simulink model "lidar_webcam_interpolation"  (Simulink 7.3)
settings: Solver=FixedStepDiscrete  StartTime=0.0  StopTime=inf  MaxStep=0.2  RelTol=1e-3
libraries: vipstatistics x1, simulink x1, dspstat3 x1, dspmtrx3 x1
settings Model: Creator=gclayton  LastModifiedBy=wildcat
settings DebuggingCC: InheritedTsInSrcMsg=none
settings RTWCC: SystemTargetFile=rlnx.tlc  GenCodeOnly=on  TemplateMakefile=rlnx_ubuntu.tmf  Description=Linux Real-Time Target  ProcessScript=rlnx_make_rtw_hook
settings RTWCC: CustomInclude=|
  | /usr/local/include/opencv/
  | /usr/local/include/
settings CodeAppCC: GenerateComments=off  SimulinkBlockComments=off
settings STFCustomTargetCC: ModelReferenceCompliant=off  MatFileLogging=on  SystemTargetFile=rlnx.tlc
settings GRTTargetCC: ModelReferenceCompliant=off  ParMdlRefBuildCompliant=off  CompOptLevelCompliant=off
settings CustomProperty: DataType=string  Value=-lm -ldl /usr/local/lib/libopencv_highgui.so.2.4 /usr/local/lib/libopencv_core.so.2.4 /usr/local/lib/libopencv_imgproc.so.2.4 -lc_urg -lc_urg_connection -lc_urg_system -lphidget21
settings EnumStrPairs: String=PC

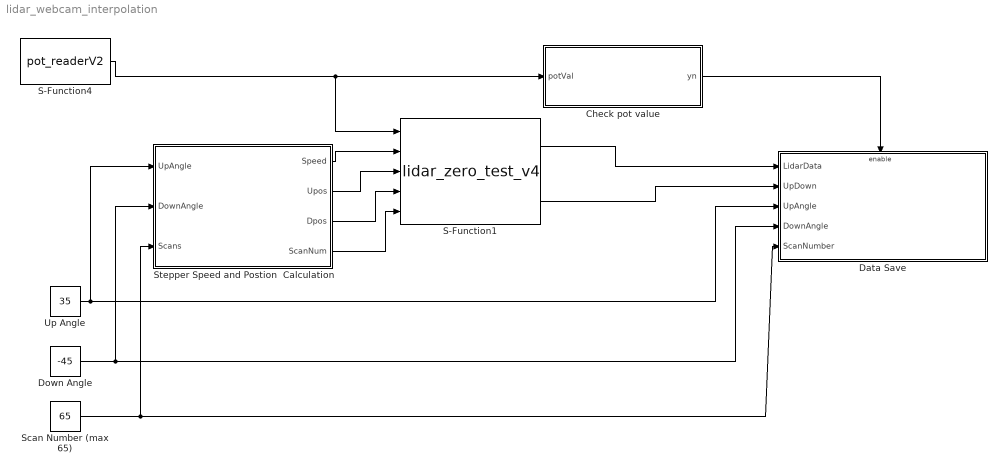
== system lidar_webcam_interpolation ==
  Check pot value : Stateflow chart  TreatAsAtomicUnit=on
  Data Save : Subsystem  TreatAsAtomicUnit=on
  Down Angle : Constant  Value=-45
  S-Function1 : S-Function  FunctionName=lidar_zero_test_v4  EnableBusSupport=off
  S-Function4 : S-Function  FunctionName=pot_readerV2  EnableBusSupport=off
  Scan Number (max 65) : Constant  Value=65
  Stepper Speed and Postion  Calculation : Stateflow chart  TreatAsAtomicUnit=on
  Up Angle : Constant  Value=35
  wires:
  S-Function4/1 -> S-Function1/1, Check pot value/1(potVal)
  Check pot value/1(yn) -> Data Save/Enable
  Scan Number (max 65)/1 -> Stepper Speed and Postion  Calculation/3(Scans), Data Save/5(ScanNumber)
  Down Angle/1 -> Stepper Speed and Postion  Calculation/2(DownAngle), Data Save/4(DownAngle)
  Up Angle/1 -> Stepper Speed and Postion  Calculation/1(UpAngle), Data Save/3(UpAngle)
  Stepper Speed and Postion  Calculation/1(Speed) -> S-Function1/2
  Stepper Speed and Postion  Calculation/2(Upos) -> S-Function1/3
  Stepper Speed and Postion  Calculation/3(Dpos) -> S-Function1/4
  Stepper Speed and Postion  Calculation/4(ScanNum) -> S-Function1/5
  S-Function1/1 -> Data Save/1(LidarData)
  S-Function1/2 -> Data Save/2(UpDown)

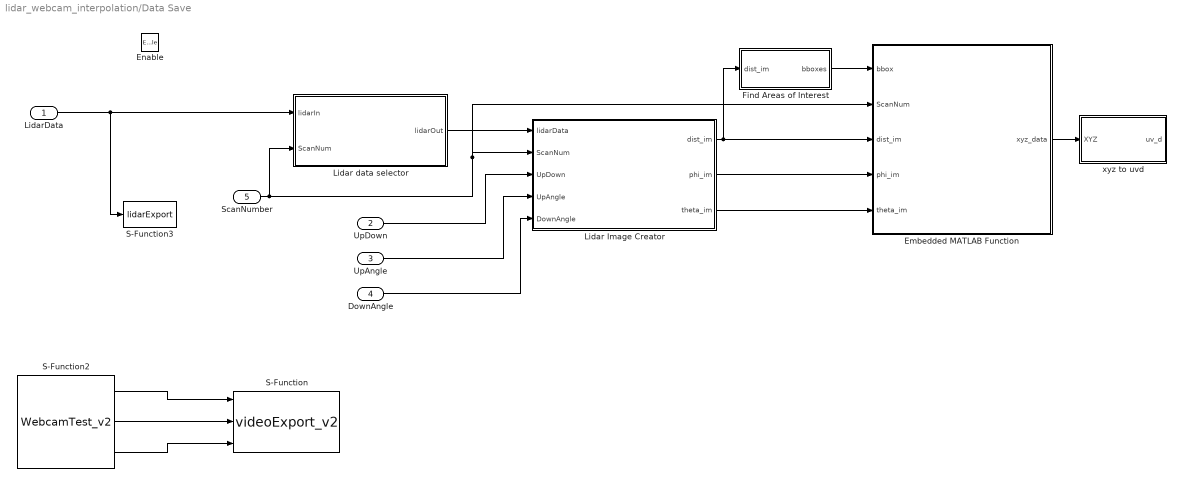
== system lidar_webcam_interpolation/Data Save ==
  LidarData : Inport
  UpDown : Inport  Port=2
  UpAngle : Inport  Port=3
  DownAngle : Inport  Port=4
  ScanNumber : Inport  Port=5
  Enable : EnablePort
  Embedded MATLAB Function : Stateflow chart  TreatAsAtomicUnit=on
  Find Areas of Interest : Subsystem
  Lidar Image Creator : Stateflow chart  TreatAsAtomicUnit=on
  Lidar data selector : Stateflow chart  TreatAsAtomicUnit=on
  S-Function : S-Function  FunctionName=videoExport_v2  EnableBusSupport=off
  S-Function2 : S-Function  FunctionName=WebcamTest_v2  EnableBusSupport=off
  S-Function3 : S-Function  FunctionName=lidarExport  EnableBusSupport=off
  xyz to uvd : Stateflow chart  TreatAsAtomicUnit=on
  wires:
  S-Function2/3 -> S-Function/3
  S-Function2/2 -> S-Function/2
  S-Function2/1 -> S-Function/1
  LidarData/1 -> S-Function3/1, Lidar data selector/1(lidarIn)
  ScanNumber/1 -> Lidar data selector/2(ScanNum), Lidar Image Creator/2(ScanNum), Embedded MATLAB Function/2(ScanNum)
  Lidar data selector/1(lidarOut) -> Lidar Image Creator/1(lidarData)
  UpDown/1 -> Lidar Image Creator/3(UpDown)
  UpAngle/1 -> Lidar Image Creator/4(UpAngle)
  DownAngle/1 -> Lidar Image Creator/5(DownAngle)
  Lidar Image Creator/1(dist_im) -> Embedded MATLAB Function/3(dist_im), Find Areas of Interest/1(dist_im)
  Lidar Image Creator/2(phi_im) -> Embedded MATLAB Function/4(phi_im)
  Lidar Image Creator/3(theta_im) -> Embedded MATLAB Function/5(theta_im)
  Find Areas of Interest/1(bboxes) -> Embedded MATLAB Function/1(bbox)
  Embedded MATLAB Function/1(xyz_data) -> xyz to uvd/1(XYZ)

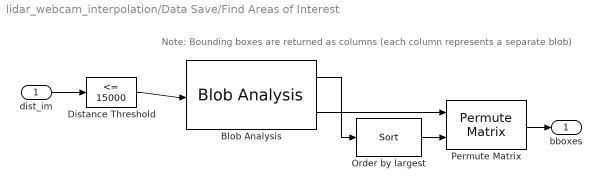
== system lidar_webcam_interpolation/Data Save/Find Areas of Interest ==
  note: Note: Bounding boxes are returned as columns (each column represents a separate blob)
  dist_im : Inport
  Blob Analysis : vipstatistics/Blob Analysis  Tag=vipblks_row_conv  area=on  centroid=off  bBox=on  majorAxis=off  minorAxis=off  angle=off  eccentricity=off  equivDiameterSq=off  extent=off  perimeter=off  maxBlobs=8  warnIfNumBlobsExceeded=on  isCount=off  useMinArea=off  minArea=0  useMaxArea=off  maxArea=intmax('uint32')  excludeBorderBlob=off  outDT=double  isOutVarDim=off  isFill=on  fillValues=-1  conn=8  isLabel=off  outputMode=Binary point scaling  outputWordLength=32  outputFracLength=16  firstCoeffMode=Binary point scaling  firstCoeffWordLength=16  firstCoeffFracLength=14  secondCoeffMode=Binary point scaling  secondCoeffWordLength=32  secondCoeffFracLength=16  accumMode=Binary point scaling  accumWordLength=32  accumFracLength=0  prodOutputMode=Binary point scaling  prodOutputWordLength=32  prodOutputFracLength=16  roundingMode=Floor  overflowMode=off
  Distance Threshold : simulink/Logic and Bit Operations/Compare To Constant  relop=<=  const=15000  OutDataTypeStr=boolean  ZeroCross=off
  Order by largest : dspstat3/Sort  otype=Index  dir=Descending  sortAlg=Quick sort  accumDataTypeStr=Inherit: Same as product output  accumLastDataTypeStr=Inherit: Same as product output  roundingMode=Floor  overflowMode=off
  Permute Matrix : dspmtrx3/Permute Matrix  mode=Columns  ZeroOneIdxMode=One-based  errmode=Clip index  checkDims=off
  bboxes : Outport
  wires:
  dist_im/1 -> Distance Threshold/1
  Distance Threshold/1 -> Blob Analysis/1
  Blob Analysis/2 -> Permute Matrix/1
  Order by largest/1 -> Permute Matrix/2
  Blob Analysis/1 -> Order by largest/1
  Permute Matrix/1 -> bboxes/1

== matlab function Stepper Speed and Postion Calculation ==
  data: UpAngle input double; Speed output double; DownAngle input double; Scans input double; Upos output double; Dpos output double; ScanNum output double
function [Speed,Upos,Dpos,ScanNum] = stepper_calc(UpAngle,DownAngle,Scans)

% This function inputs desired positive and negative scan angles
% and desired number of scans and outputs results positions for
% the stepper and the required speed of the stepper motor to properly
% move so the desired number of scans is obtained over the course of
% the motion of the stepper

% Scan Number requires no change
ScanNum = Scans;

% Transformation of angle to stepper position obtained from stepper calibration
% Output must be an integer
% 57 is added or subtracted due to wobble of gimbal system
Upos = round(UpAngle*1036/45)-57;
Dpos = round(DownAngle*1036/45)+57;

% Transformation of speed based 
% Output must be an interger
Speed = round(abs(UpAngle-DownAngle) * (1214/90) * 65/Scans);

== matlab function Check pot value ==
  data: potVal input double; yn output double
function yn = check_pot_val(potVal)
%#eml

% Pot value may initially be zero.
% Check for this and output a 1 or zero to 
% control whether the rest of model runs
if (potVal == 0)
    yn = 0;
else
    yn = 1;
end

== matlab function Data Save/Lidar data selector ==
  data: lidarIn input double; lidarOut output double; ScanNum input double
function lidarOut = data_selector(lidarIn,ScanNum)
% Lidar data is always input as a 1x70200 matrix.
% If Scan Number is less than 65 some of this data may be blank
% Select only the parts of the matrix where data has been collected
DataLength = 1080*ScanNum;
lidarOut = zeros(1,DataLength);

for i=1:DataLength
    if (lidarIn(i)<2)
        lidarIn(i) = 30000;
    end
    lidarOut(i) = lindarIn(i);
end

% indexes = 1:70200;
% lidarOut = lidarIn(indexes);

== matlab function Data Save/Lidar Image Creator ==
  data: lidarData input double; ScanNum input double; dist_im output double; phi_im output double; theta_im output double; UpDown input double; UpAngle input double; DownAngle input double
function [dist_im, phi_im, theta_im] = image_creator(lidarData,ScanNum,UpDown,UpAngle,DownAngle)
%#eml

% Define variables based on gimbal system and scan pattern
DataLength = 1080*ScanNum;
h = 36.3;

% Define Data sizes
phim = zeros(1,DataLength);
thetam = zeros(1,DataLength);
distm = zeros(1,DataLength);
dist_im = zeros(ScanNum,540);
phi_im = zeros(ScanNum,540);
theta_im = zeros(ScanNum,540);


%Define phi_rad: angles corresponding to one lidar scan
l = 1:1080;
phi_rad = (-45 + 0.25*l)*pi/180;

% Repeat phim for number of scans
for i = 1:ScanNum
        
    for j = 1 : 1080
        phi_val = 1080*(i-1) + j;
        phim(1,phi_val) = phi_rad(1,j);
    end
end

% Theta changes from -45 to 45 degrees over the duration of the scan
theta_min = DownAngle*pi/180;
theta_max = UpAngle*pi/180;
theta_step = (theta_max - theta_min)/DataLength;
if (UpDown == 0)
    thetam = [theta_max : -theta_step : (theta_min+theta_step)];
elseif (UpDown == 1)
    thetam = [theta_min : theta_step : (theta_max-theta_step)];
end

% Distance matrix is directly from lidar data
distm = lidarData';


% Create images for distance, phi, and theta
for i2 = 1:ScanNum
    for j2 = 1:540
        dist_im(i2,j2) = distm(1, 270+j2 + 1080*(i2-1));
        phi_im(i2,j2) = phim(1, 270+j2 + 1080*(i2-1));
        theta_im(i2,j2) = thetam(1, 270+j2 + 1080*(i2-1));
    end
    
end

== matlab function Data Save/Embedded MATLAB Function ==
  data: bbox input double; xyz_data output double; ScanNum input double; dist_im input double; phi_im input double; theta_im input double
function xyz_data  = fcn(bbox,ScanNum,dist_im,phi_im,theta_im)
% Generate x,y,z data from images found using blob analysis

h = 36.3;


bbox_size = size(bbox);
box_num = bbox_size(1);

x_bbox = bbox(:,1);
y_bbox = bbox(:,2);
w_bbox = bbox(:,3);
h_bbox = bbox(:,4);

max_w = w_bbox(1);
max_h = h_bbox(1);

M = (max_w+2)*(max_h+2);
xyz_data = zeros(M,3,box_num);
xd = zeros(max_h+2,max_w+2);
yd = zeros(max_h+2,max_w+2);
zd = zeros(max_h+2,max_w+2);

% Reapeat for number of bounding boxes
for i = 1:box_num
    % Find x and y position of current bounding box
    x_pos = x_bbox(i);
    y_pos = y_bbox(i);
    
    % Find minimum and maximum positions to look for in bounding boxes
    % Limit x and y range to being within image frame (ScanNum x 540)
    x_min = round(x_pos - 0.5*max_h) - 2;
    if (x_min < 1)
        x_min = 1;
    end
    
    x_max = round(x_pos + 0.5*max_h) + 2;
    if (x_max > ScanNum)
        x_max = ScanNum;
    end
    
    y_min = round(y_pos - 0.5*max_w) - 2;
    if (y_min < 1)
        y_min = 1;
    end
    
    y_max = round(y_pos + 0.5*max_w) + 2;
    if (y_max > 540)
        y_max = 540;
    end
    
    % Find length of x vector for placing values in xyz_data
    x_length = x_max-x_min;
    
    % Find x y and z data within each of the boxes
    % The three images have corresponding values for distance theta and phi at each position
    for j = x_min:x_max
        for k = y_min:y_max
            xd(j,k) = dist_im(j,k)*cos(j,k);
            yd(j,k) = dist_im(j,k)*sin(phi_im(j,k))*cos(theta_im(j,k)) - h*sin(theta_im(j,k));
            zd(j,k) = dist_im(j,k)*sin(phi_im(j,k))*sin(theta_im(j,k)) + h*cos(theta_im(j,l));
            
            % Put x y and z into corresponding section in xyz_data
            % k + x_length*(j-1) is the M loction
            xyz_data(k + x_length*(j-1), 1, i) = xd(j,k);
            xyz_data(k + x_length*(j-1), 2, i) = yd(j,k);
            xyz_data(k + x_length*(j-1), 3, i) = zd(j,k);
            
            
            %xd(i,j) = distm(i,j)*cos(phim(i,j));
            %yd(i,j) = distm(i,j)*sin(phim(i,j))*cos(thetam(i,j)) - h*sin(thetam(i,j));
            %zd(i,j) = distm(i,j)*sin(phim(i,j))*sin(thetam(i,j)) + h*cos(thetam(i,j));
            
        end
    end
end

== matlab function Data Save/xyz to uvd ==
  data: XYZ input double; uv_d output double
function uv_d = xyz2uv(XYZ)
%Written by Anderson Lebbad on July 2, 2014
%Last Edited:
%
%This function transforms a Mx3xN array of points (where M is the maximum
%number of points contained within an individual blob bbox, the three
%columns represent x, y, and z respectively, and N is the number of blobs -
%set to 8 currently) into the uv frame of the camera.

%% Analyze input and set size of transformation output

[M,~,N] = size(XYZ);
beyondRange = 30000;
uv_d = beyondRange*ones(480,640);

%% Set Variables

% Translation vector (in millimeters)
t = [24; -113; 38];

% Rotation angles
phi = (-90+6)*pi/180;
theta = 0*pi/180;

% Rotation about the x-axis
Rx = [1 0 0; 0 cos(phi) sin(phi); 0 -sin(phi) cos(phi)];
% Followed by rotation about the y-axis
R = [cos(theta) 0 -sin(theta); 0 1 0; sin(theta) 0 cos(theta)]*Rx;

% Transformation matrix
T = [R t];

% Radial Distortions
RadDist = [0.069102182282360,-0.154608606024690,0.020241053576861];

% Intrinsic Matrix
K = [5.548581600685270e+02,0,0;0,5.523116000564020e+02,0;3.135858904821101e+02,2.190392333699872e+02,1];
KK = K';

%% Loop for multiple blobs

for i=1:N
    % Remove null points
    numNull = sum(XYZ(:,2,i) == -1);
    X = XYZ(1:M-numNull,1,i);
    Y = XYZ(1:M-numNull,2,i);
    Z = XYZ(1:M-numNull,3,i);
    
    % Transformation
    Xc = T(1,1)*X+T(1,2)*Y+T(1,3)*Z+T(1,4);
    Yc = T(2,1)*X+T(2,2)*Y+T(2,3)*Z+T(2,4);
    Zc = T(3,1)*X+T(3,2)*Y+T(3,3)*Z+T(3,4);
    
    % Normalize Coordinates
    Xn = Xc./Zc;
    Yn = Yc./Zc;
    % Calculate Distance to each point from camera
    Dp = sqrt(Xc.^2+Yc.^2+Zc.^2);
    
    % Radial Vectors
    r2 = Xn.^2+Yn.^2;
    r6 = r2.^3;
    % Distorted Coodinates
    Xd = Xn.*(1+RadDist(1).*r2+RadDist(3).*r6);
    Yd = Yn.*(1+RadDist(1).*r2+RadDist(3).*r6);
    
    % Pixel Coordinates
    Xp = KK(1,1)*Xd+KK(1,2)*Yd+KK(1,3);
    Yp = KK(2,1)*Xd+KK(2,2)*Yd+KK(2,3);
    
    % Find area the blob is bound by in the image coordinates
    minX = ceil(min(Xp));
    maxX = floor(max(Xp));
    minY = ceil(min(Yp));
    maxY = floor(max(Yp));
    
    % Check to make sure blob is (at least partially) within image frame
    if (minX < 640) && (maxX > 1) && (minY < 480) && (maxY > 1)
        
        % Set interpolation vectors to not exceed frame
        minX = max(minX,1);
        maxX = min(maxX,640);
        minY = max(minY,1);
        maxY = min(maxY,480);
        numX = maxX-minX+1;
        numY = maxY-minY+1;
        uvdPts = zeros(numY,numX);
        
        % Run interpolation over bounded region
        for j = 1:numX
            for k = 1:numY
                % L1 Norm for nearest neighbor interpolation
                [~,I] = min(abs(Xp-j)+abs(Yp-k));
                % Assign index values into pointer array
                uvdPts(k,j) = I(1);
            end
        end
        % Use pointer array to assign depth values into output frame
        uv_d(minY:maxY,minX:maxX) = Dp(uvdPts);
    end
end

end
